simulink model "Step_12_TheEstimatedINVDynamicsMatricesCTC"  (R2020a)
settings: Solver=ode4  StartTime=0.0  StopTime=10  FixedStep=2e-3  RelTol=1e-3
model workspace (MATLAB code in the model file):
  | dhparams = [0   0   0.6   0;
  |             0   0   0     pi/2;
  |             0   0   0.5   0];
  | 
  | rrrRobot = rigidBodyTree('DataFormat', 'column', 'MaxNumBodies', 4);
  | 
  | bodyNames = {'link1', 'link2', 'link3'};
  | jointNames = {'joint1', 'joint2', 'joint3'};
  | parentNames = {'base', 'link1', 'link2'};
  | 
  | for i = 1:3
  |     body = rigidBody(bodyNames{i});
  |     joint = rigidBodyJoint(jointNames{i}, 'revolute');
  |     setFixedTransform(joint, dhparams(i,:), 'dh');
  |     body.Joint = joint;
  |     addBody(rrrRobot, body, parentNames{i});
  | end
  | 
  | tool = rigidBody('tool');
  | jointTool = rigidBodyJoint('fix_tip', 'fixed');
  | setFixedTransform(jointTool, eye(4));
  | tool.Joint = jointTool;
  | addBody(rrrRobot, tool, 'link3');
undefined symbols (not defined in the file or in its folder): X, Y, Z
libraries: sm_lib x34, nesl_utility x10
(part 2 of 2)

== matlab function Step_12_TheEstimatedINVDynamicsMatricesCTC/CTC/Estimated_C ==
  data: Q input; EstTau_C output; Qp input
function EstTau_C = Estimated_C(Q,Qp)
%#codegen

%    This function was generated by the Symbolic Math Toolbox version 8.5.
%    10-Jul-2026 17:57:50

q1 = Q(1,:);
q2 = Q(2,:);
q3 = Q(3,:);
qp1 = Qp(1,:);
qp2 = Qp(2,:);
qp3 = Qp(3,:);
EstTau_C = [qp1.*8.650376988596507e-4+tanh(qp1.*1.0e+2).*2.609157356257976e-3+cos(q2+q3).*(sin(q1).*(qp1.*qp2.*cos(q1)+qp1.*qp3.*cos(q1))-cos(q1).*(qp1.*qp2.*sin(q1)+qp1.*qp3.*sin(q1))).*2.289775576171808e-3-(qp2.*cos(q1).^2.*sin(q2)+qp2.*sin(q1).^2.*sin(q2)).*(qp2.*cos(q1).^2+qp2.*sin(q1).^2).*1.139509685512077e-2+(cos(q2+q3).*cos(q1).*(qp2.*cos(q1)+qp3.*cos(q1))+cos(q2+q3).*sin(q1).*(qp2.*sin(q1)+qp3.*sin(q1))).*(qp1.*cos(q2+q3)+sin(q2+q3).*sin(q1).*(qp2.*cos(q1)+qp3.*cos(q1))-sin(q2+q3).*cos(q1).*(qp2.*sin(q1)+qp3.*sin(q1))).*7.317250181898908e-3-sin(q2+q3).*(sin(q1).*(qp1.*qp2.*cos(q1)+qp1.*qp3.*cos(q1))-cos(q1).*(qp1.*qp2.*sin(q1)+qp1.*qp3.*sin(q1))).*5.967026219736011e-3-(sin(q2+q3).*cos(q1).*(qp2.*cos(q1)+qp3.*cos(q1))+sin(q2+q3).*sin(q1).*(qp2.*sin(q1)+qp3.*sin(q1))).*(qp1.*sin(q2+q3)-cos(q2+q3).*sin(q1).*(qp2.*cos(q1)+qp3.*cos(q1))+cos(q2+q3).*cos(q1).*(qp2.*sin(q1)+qp3.*sin(q1))).*7.317250181898908e-3+cos(q2+q3).*((cos(q1).*cos(q2).*(qp1.*qp2.*cos(q1)+qp1.*qp3.*cos(q1)))./2.0+(cos(q2).*sin(q1).*(qp1.*qp2.*sin(q1)+qp1.*qp3.*sin(q1)))./2.0+(qp1.*cos(q1).*cos(q2).*(qp2.*cos(q1)+qp3.*cos(q1)))./2.0+(qp1.*cos(q2).*sin(q1).*(qp2.*sin(q1)+qp3.*sin(q1)))./2.0).*3.199478300720183e-7+cos(q2).*(qp1.*qp2.*cos(q1).^2.*cos(q2)+qp1.*qp2.*cos(q2).*sin(q1).^2).*3.327734875462438e-3-(sin(q2+q3).*cos(q1).*(qp2.*cos(q1)+qp3.*cos(q1))+sin(q2+q3).*sin(q1).*(qp2.*sin(q1)+qp3.*sin(q1))).*(qp1.*cos(q2+q3)+sin(q2+q3).*sin(q1).*(qp2.*cos(q1)+qp3.*cos(q1))-sin(q2+q3).*cos(q1).*(qp2.*sin(q1)+qp3.*sin(q1))).*6.62632259505323e-2-(sin(q1).*(qp2.*sin(q1)+qp3.*sin(q1))+cos(q1).*(qp2.*cos(q1)+qp3.*cos(q1))).*(cos(q2+q3).*cos(q1).*(qp2.*cos(q1)+qp3.*cos(q1))+cos(q2+q3).*sin(q1).*(qp2.*sin(q1)+qp3.*sin(q1))).*5.967026219736011e-3-sin(q2+q3).*((cos(q1).*cos(q2).*(qp1.*qp2.*cos(q1)+qp1.*qp3.*cos(q1)))./2.0+(cos(q2).*sin(q1).*(qp1.*qp2.*sin(q1)+qp1.*qp3.*sin(q1)))./2.0+(qp1.*cos(q1).*cos(q2).*(qp2.*cos(q1)+qp3.*cos(q1)))./2.0+(qp1.*cos(q2).*sin(q1).*(qp2.*sin(q1)+qp3.*sin(q1)))./2.0).*3.000177417317213e-1+sin(q2).*(qp1.*qp2.*cos(q1).^2.*cos(q2)+qp1.*qp2.*cos(q2).*sin(q1).^2).*1.801758335412092e-2-cos(q2).*(qp1.*qp2.*cos(q1).^2.*sin(q2)+qp1.*qp2.*sin(q1).^2.*sin(q2)).*5.794502385359621e-1+cos(q2+q3).*(cos(q2+q3).*cos(q1).*(qp1.*qp2.*cos(q1)+qp1.*qp3.*cos(q1))+cos(q2+q3).*sin(q1).*(qp1.*qp2.*sin(q1)+qp1.*qp3.*sin(q1))).*7.317250181898908e-3-(sin(q1).*(qp2.*sin(q1)+qp3.*sin(q1))+cos(q1).*(qp2.*cos(q1)+qp3.*cos(q1))).*(sin(q2+q3).*cos(q1).*(qp2.*cos(q1)+qp3.*cos(q1))+sin(q2+q3).*sin(q1).*(qp2.*sin(q1)+qp3.*sin(q1))).*2.289775576171808e-3-sin(q2).*(qp1.*qp2.*cos(q1).^2.*sin(q2)+qp1.*qp2.*sin(q1).^2.*sin(q2)).*3.327734875462438e-3-cos(q2+q3).*(sin(q2+q3).*cos(q1).*(qp1.*qp2.*cos(q1)+qp1.*qp3.*cos(q1))+sin(q2+q3).*sin(q1).*(qp1.*qp2.*sin(q1)+qp1.*qp3.*sin(q1))).*6.62632259505323e-2-sin(q2+q3).*(sin(q2+q3).*cos(q1).*(qp1.*qp2.*cos(q1)+qp1.*qp3.*cos(q1))+sin(q2+q3).*sin(q1).*(qp1.*qp2.*sin(q1)+qp1.*qp3.*sin(q1))).*7.317250181898908e-3-(sin(q1).*(qp2.*cos(q1)+qp3.*cos(q1))-cos(q1).*(qp2.*sin(q1)+qp3.*sin(q1))).*(qp1.*sin(q2+q3)-cos(q2+q3).*sin(q1).*(qp2.*cos(q1)+qp3.*cos(q1))+cos(q2+q3).*cos(q1).*(qp2.*sin(q1)+qp3.*sin(q1))).*5.967026219736011e-3+(sin(q1).*(qp2.*cos(q1)+qp3.*cos(q1))-cos(q1).*(qp2.*sin(q1)+qp3.*sin(q1))).*(qp1.*cos(q2+q3)+sin(q2+q3).*sin(q1).*(qp2.*cos(q1)+qp3.*cos(q1))-sin(q2+q3).*cos(q1).*(qp2.*sin(q1)+qp3.*sin(q1))).*2.289775576171808e-3+(sin(q1).*(qp2.*sin(q1)+qp3.*sin(q1))+cos(q1).*(qp2.*cos(q1)+qp3.*cos(q1))).*(sin(q1).*(qp2.*cos(q1)+qp3.*cos(q1))-cos(q1).*(qp2.*sin(q1)+qp3.*sin(q1))).*8.244272995860623e-2+(qp2.*cos(q1).^2.*cos(q2)+qp2.*cos(q2).*sin(q1).^2).*(qp2.*cos(q1).^2+qp2.*sin(q1).^2).*7.881605381698013e-5-cos(q2+q3).*cos(q1).*(qp1.*((qp1.*cos(q2).*sin(q1))./2.0+(qp2.*cos(q1).*sin(q2))./2.0)+qp2.*((qp1.*cos(q1).*sin(q2))./2.0+(qp2.*cos(q2).*sin(q1))./2.0)-(qp2.*cos(q1)+qp3.*cos(q1)).*((cos(q2).*sin(q1).*(qp2.*cos(q1)+qp3.*cos(q1)))./2.0-(cos(q1).*cos(q2).*(qp2.*sin(q1)+qp3.*sin(q1)))./2.0)-(qp1.^2.*cos(q2).*sin(q1))./2.0).*3.000177417317213e-1-sin(q2+q3).*cos(q1).*(qp1.*((qp1.*cos(q2).*sin(q1))./2.0+(qp2.*cos(q1).*sin(q2))./2.0)+qp2.*((qp1.*cos(q1).*sin(q2))./2.0+(qp2.*cos(q2).*sin(q1))./2.0)-(qp2.*cos(q1)+qp3.*cos(q1)).*((cos(q2).*sin(q1).*(qp2.*cos(q1)+qp3.*cos(q1)))./2.0-(cos(q1).*cos(q2).*(qp2.*sin(q1)+qp3.*sin(q1)))./2.0)-(qp1.^2.*cos(q2).*sin(q1))./2.0).*3.199478300720183e-7+cos(q2+q3).*sin(q1).*((qp2.*sin(q1)+qp3.*sin(q1)).*((cos(q2).*sin(q1).*(qp2.*cos(q1)+qp3.*cos(q1)))./2.0-(cos(q1).*cos(q2).*(qp2.*sin(q1)+qp3.*sin(q1)))./2.0)+qp1.*((qp1.*cos(q1).*cos(q2))./2.0-(qp2.*sin(q1).*sin(q2))./2.0)+qp2.*((qp2.*cos(q1).*cos(q2))./2.0-(qp1.*sin(q1).*sin(q2))./2.0)-(qp1.^2.*cos(q1).*cos(q2))./2.0).*3.000177417317213e-1+qp1.*cos(q2).*(qp2.*cos(q1).^2.*cos(q2)+qp2.*cos(q2).*sin(q1).^2).*3.327734875462438e-3+sin(q2+q3).*sin(q1).*((qp2.*sin(q1)+qp3.*sin(q1)).*((cos(q2).*sin(q1).*(qp2.*cos(q1)+qp3.*cos(q1)))./2.0-(cos(q1).*cos(q2).*(qp2.*sin(q1)+qp3.*sin(q1)))./2.0)+qp1.*((qp1.*cos(q1).*cos(q2))./2.0-(qp2.*sin(q1).*sin(q2))./2.0)+qp2.*((qp2.*cos(q1).*cos(q2))./2.0-(qp1.*sin(q1).*sin(q2))./2.0)-(qp1.^2.*cos(q1).*cos(q2))./2.0).*3.199478300720183e-7+qp1.*sin(q2).*(qp2.*cos(q1).^2.*cos(q2)+qp2.*cos(q2).*sin(q1).^2).*1.801758335412092e-2-qp1.*cos(q2).*(qp2.*cos(q1).^2.*sin(q2)+qp2.*sin(q1).^2.*sin(q2)).*5.794502385359621e-1-qp1.*sin(q2).*(qp2.*cos(q1).^2.*sin(q2)+qp2.*sin(q1).^2.*sin(q2)).*3.327734875462438e-3;qp2.*(-1.309534126070689e-2)+tanh(qp2.*1.0e+2).*5.718358826714878e-3-sin(q1).*((cos(q2+q3).*(qp2.*cos(q1)+qp3.*cos(q1))-qp1.*sin(q2+q3).*sin(q1)).*(qp1.*cos(q2+q3)+sin(q2+q3).*sin(q1).*(qp2.*cos(q1)+qp3.*cos(q1))-sin(q2+q3).*cos(q1).*(qp2.*sin(q1)+qp3.*sin(q1)))-sin(q2+q3).*cos(q1).*(sin(q2+q3).*cos(q1).*(qp1.*qp2.*cos(q1)+qp1.*qp3.*cos(q1))+sin(q2+q3).*sin(q1).*(qp1.*qp2.*sin(q1)+qp1.*qp3.*sin(q1)))).*6.62632259505323e-2-sin(q1).*(-(sin(q1).*(qp2.*sin(q1)+qp3.*sin(q1))+cos(q1).*(qp2.*cos(q1)+qp3.*cos(q1))).*(sin(q2+q3).*(qp2.*cos(q1)+qp3.*cos(q1))+qp1.*cos(q2+q3).*sin(q1))+sin(q1).*(cos(q2+q3).*cos(q1).*(qp1.*qp2.*cos(q1)+qp1.*qp3.*cos(q1))+cos(q2+q3).*sin(q1).*(qp1.*qp2.*sin(q1)+qp1.*qp3.*sin(q1)))+qp1.*cos(q1).*(qp1.*sin(q2+q3)-cos(q2+q3).*sin(q1).*(qp2.*cos(q1)+qp3.*cos(q1))+cos(q2+q3).*cos(q1).*(qp2.*sin(q1)+qp3.*sin(q1)))+cos(q2+q3).*cos(q1).*(sin(q1).*(qp1.*qp2.*cos(q1)+qp1.*qp3.*cos(q1))-cos(q1).*(qp1.*qp2.*sin(q1)+qp1.*qp3.*sin(q1)))).*5.967026219736011e-3-cos(q1).*(-cos(q1).*(qp1.*qp2.*cos(q1).^2.*cos(q2)+qp1.*qp2.*cos(q2).*sin(q1).^2)+(qp1.*cos(q1).*cos(q2)-qp2.*sin(q1).*sin(q2)).*(qp2.*cos(q1).^2+qp2.*sin(q1).^2)+qp1.^2.*sin(q1).*sin(q2)).*7.881605381698013e-5+cos(q2+q3).*((qp2.*sin(q1)+qp3.*sin(q1)).*((cos(q2).*(qp2.*sin(q1)+qp3.*sin(q1)))./2.0+(qp1.*cos(q1).*sin(q2))./2.0)-cos(q1).*(qp1.*((qp1.*cos(q1).*cos(q2))./2.0-(qp2.*sin(q1).*sin(q2))./2.0)+qp2.*((qp2.*cos(q1).*cos(q2))./2.0-(qp1.*sin(q1).*sin(q2))./2.0))-sin(q1).*(qp1.*((qp1.*cos(q2).*sin(q1))./2.0+(qp2.*cos(q1).*sin(q2))./2.0)+qp2.*((qp1.*cos(q1).*sin(q2))./2.0+(qp2.*cos(q2).*sin(q1))./2.0))+(qp2.*cos(q1)+qp3.*cos(q1)).*((cos(q2).*(qp2.*cos(q1)+qp3.*cos(q1)))./2.0-(qp1.*sin(q1).*sin(q2))./2.0)-(sin(q1).*sin(q2).*(qp1.*qp2.*cos(q1)+qp1.*qp3.*cos(q1)))./2.0+(cos(q1).*sin(q2).*(qp1.*qp2.*sin(q1)+qp1.*qp3.*sin(q1)))./2.0).*3.199478300720183e-7+cos(q1).*((cos(q2+q3).*(qp2.*sin(q1)+qp3.*sin(q1))+qp1.*sin(q2+q3).*cos(q1)).*(qp1.*cos(q2+q3)+sin(q2+q3).*sin(q1).*(qp2.*cos(q1)+qp3.*cos(q1))-sin(q2+q3).*cos(q1).*(qp2.*sin(q1)+qp3.*sin(q1)))-sin(q2+q3).*sin(q1).*(sin(q2+q3).*cos(q1).*(qp1.*qp2.*cos(q1)+qp1.*qp3.*cos(q1))+sin(q2+q3).*sin(q1).*(qp1.*qp2.*sin(q1)+qp1.*qp3.*sin(q1)))).*6.62632259505323e-2-cos(q1).*((sin(q1).*(qp2.*sin(q1)+qp3.*sin(q1))+cos(q1).*(qp2.*cos(q1)+qp3.*cos(q1))).*(sin(q2+q3).*(qp2.*sin(q1)+qp3.*sin(q1))-qp1.*cos(q2+q3).*cos(q1))+cos(q1).*(cos(q2+q3).*cos(q1).*(qp1.*qp2.*cos(q1)+qp1.*qp3.*cos(q1))+cos(q2+q3).*sin(q1).*(qp1.*qp2.*sin(q1)+qp1.*qp3.*sin(q1)))-qp1.*sin(q1).*(qp1.*sin(q2+q3)-cos(q2+q3).*sin(q1).*(qp2.*cos(q1)+qp3.*cos(q1))+cos(q2+q3).*cos(q1).*(qp2.*sin(q1)+qp3.*sin(q1)))-cos(q2+q3).*sin(q1).*(sin(q1).*(qp1.*qp2.*cos(q1)+qp1.*qp3.*cos(q1))-cos(q1).*(qp1.*qp2.*sin(q1)+qp1.*qp3.*sin(q1)))).*5.967026219736011e-3-cos(q1).*(-(qp1.*cos(q1).*sin(q2)+qp2.*cos(q2).*sin(q1)).*(qp2.*cos(q1).^2+qp2.*sin(q1).^2)+cos(q1).*(qp1.*qp2.*cos(q1).^2.*sin(q2)+qp1.*qp2.*sin(q1).^2.*sin(q2))+qp1.^2.*cos(q2).*sin(q1)).*1.139509685512077e-2+sin(q1).*(sin(q1).*(qp1.*qp2.*cos(q1).^2.*cos(q2)+qp1.*qp2.*cos(q2).*sin(q1).^2)-(qp1.*cos(q2).*sin(q1)+qp2.*cos(q1).*sin(q2)).*(qp2.*cos(q1).^2+qp2.*sin(q1).^2)+qp1.^2.*cos(q1).*sin(q2)).*7.881605381698013e-5-sin(q2+q3).*((qp2.*sin(q1)+qp3.*sin(q1)).*((cos(q2).*(qp2.*sin(q1)+qp3.*sin(q1)))./2.0+(qp1.*cos(q1).*sin(q2))./2.0)-cos(q1).*(qp1.*((qp1.*cos(q1).*cos(q2))./2.0-(qp2.*sin(q1).*sin(q2))./2.0)+qp2.*((qp2.*cos(q1).*cos(q2))./2.0-(qp1.*sin(q1).*sin(q2))./2.0))-sin(q1).*(qp1.*((qp1.*cos(q2).*sin(q1))./2.0+(qp2.*cos(q1).*sin(q2))./2.0)+qp2.*((qp1.*cos(q1).*sin(q2))./2.0+(qp2.*cos(q2).*sin(q1))./2.0))+(qp2.*cos(q1)+qp3.*cos(q1)).*((cos(q2).*(qp2.*cos(q1)+qp3.*cos(q1)))./2.0-(qp1.*sin(q1).*sin(q2))./2.0)-(sin(q1).*sin(q2).*(qp1.*qp2.*cos(q1)+qp1.*qp3.*cos(q1)))./2.0+(cos(q1).*sin(q2).*(qp1.*qp2.*sin(q1)+qp1.*qp3.*sin(q1)))./2.0).*3.000177417317213e-1-sin(q1).*(qp1.*cos(q2).*(qp1.*cos(q2).*sin(q1)+qp2.*cos(q1).*sin(q2))+cos(q1).*sin(q2).*(qp1.*qp2.*cos(q1).^2.*cos(q2)+qp1.*qp2.*cos(q2).*sin(q1).^2)+qp1.*sin(q2).*(qp2.*cos(q1).*cos(q2)-qp1.*sin(q1).*sin(q2))+cos(q1).*cos(q2).*(qp1.*qp2.*cos(q1).^2.*sin(q2)+qp1.*qp2.*sin(q1).^2.*sin(q2))).*3.327734875462438e-3-sin(q1).*((sin(q2+q3).*(qp2.*cos(q1)+qp3.*cos(q1))+qp1.*cos(q2+q3).*sin(q1)).*(qp1.*cos(q2+q3)+sin(q2+q3).*sin(q1).*(qp2.*cos(q1)+qp3.*cos(q1))-sin(q2+q3).*cos(q1).*(qp2.*sin(q1)+qp3.*sin(q1)))+(cos(q2+q3).*(qp2.*cos(q1)+qp3.*cos(q1))-qp1.*sin(q2+q3).*sin(q1)).*(qp1.*sin(q2+q3)-cos(q2+q3).*sin(q1).*(qp2.*cos(q1)+qp3.*cos(q1))+cos(q2+q3).*cos(q1).*(qp2.*sin(q1)+qp3.*sin(q1)))+sin(q2+q3).*cos(q1).*(cos(q2+q3).*cos(q1).*(qp1.*qp2.*cos(q1)+qp1.*qp3.*cos(q1))+cos(q2+q3).*sin(q1).*(qp1.*qp2.*sin(q1)+qp1.*qp3.*sin(q1)))+cos(q2+q3).*cos(q1).*(sin(q2+q3).*cos(q1).*(qp1.*qp2.*cos(q1)+qp1.*qp3.*cos(q1))+sin(q2+q3).*sin(q1).*(qp1.*qp2.*sin(q1)+qp1.*qp3.*sin(q1)))).*7.317250181898908e-3-sin(q1).*((qp2.*cos(q1).*cos(q2)-qp1.*sin(q1).*sin(q2)).*(qp2.*cos(q1).^2+qp2.*sin(q1).^2)+sin(q1).*(qp1.*qp2.*cos(q1).^2.*sin(q2)+qp1.*qp2.*sin(q1).^2.*sin(q2))-qp1.^2.*cos(q1).*cos(q2)).*1.139509685512077e-2+cos(q2+q3).*cos(q1).^2.*2.940173868970869+cos(q1).*(-qp1.*cos(q2).*(qp1.*cos(q1).*cos(q2)-qp2.*sin(q1).*sin(q2))+qp1.*sin(q2).*(qp1.*cos(q1).*sin(q2)+qp2.*cos(q2).*sin(q1))+sin(q1).*sin(q2).*(qp1.*qp2.*cos(q1).^2.*cos(q2)+qp1.*qp2.*cos(q2).*sin(q1).^2)+cos(q2).*sin(q1).*(qp1.*qp2.*cos(q1).^2.*sin(q2)+qp1.*qp2.*sin(q1).^2.*sin(q2))).*3.327734875462438e-3+cos(q2+q3).*sin(q1).^2.*2.940173868970869+sin(q2+q3).*cos(q1).^2.*3.135488734705779e-6-sin(q1).*((sin(q1).*(qp2.*sin(q1)+qp3.*sin(q1))+cos(q1).*(qp2.*cos(q1)+qp3.*cos(q1))).*(cos(q2+q3).*(qp2.*cos(q1)+qp3.*cos(q1))-qp1.*sin(q2+q3).*sin(q1))+sin(q1).*(sin(q2+q3).*cos(q1).*(qp1.*qp2.*cos(q1)+qp1.*qp3.*cos(q1))+sin(q2+q3).*sin(q1).*(qp1.*qp2.*sin(q1)+qp1.*qp3.*sin(q1)))-qp1.*cos(q1).*(qp1.*cos(q2+q3)+sin(q2+q3).*sin(q1).*(qp2.*cos(q1)+qp3.*cos(q1))-sin(q2+q3).*cos(q1).*(qp2.*sin(q1)+qp3.*sin(q1)))+sin(q2+q3).*cos(q1).*(sin(q1).*(qp1.*qp2.*cos(q1)+qp1.*qp3.*cos(q1))-cos(q1).*(qp1.*qp2.*sin(q1)+qp1.*qp3.*sin(q1)))).*2.289775576171808e-3+sin(q2+q3).*sin(q1).^2.*3.135488734705779e-6+cos(q1).*((sin(q1).*(qp2.*sin(q1)+qp3.*sin(q1))+cos(q1).*(qp2.*cos(q1)+qp3.*cos(q1))).*(cos(q2+q3).*(qp2.*sin(q1)+qp3.*sin(q1))+qp1.*sin(q2+q3).*cos(q1))-cos(q1).*(sin(q2+q3).*cos(q1).*(qp1.*qp2.*cos(q1)+qp1.*qp3.*cos(q1))+sin(q2+q3).*sin(q1).*(qp1.*qp2.*sin(q1)+qp1.*qp3.*sin(q1)))+sin(q2+q3).*sin(q1).*(sin(q1).*(qp1.*qp2.*cos(q1)+qp1.*qp3.*cos(q1))-cos(q1).*(qp1.*qp2.*sin(q1)+qp1.*qp3.*sin(q1)))-qp1.*sin(q1).*(qp1.*cos(q2+q3)+sin(q2+q3).*sin(q1).*(qp2.*cos(q1)+qp3.*cos(q1))-sin(q2+q3).*cos(q1).*(qp2.*sin(q1)+qp3.*sin(q1)))).*2.289775576171808e-3+cos(q1).*((cos(q2+q3).*(qp2.*sin(q1)+qp3.*sin(q1))+qp1.*sin(q2+q3).*cos(q1)).*(qp1.*sin(q2+q3)-cos(q2+q3).*sin(q1).*(qp2.*cos(q1)+qp3.*cos(q1))+cos(q2+q3).*cos(q1).*(qp2.*sin(q1)+qp3.*sin(q1)))+(sin(q2+q3).*(qp2.*sin(q1)+qp3.*sin(q1))-qp1.*cos(q2+q3).*cos(q1)).*(qp1.*cos(q2+q3)+sin(q2+q3).*sin(q1).*(qp2.*cos(q1)+qp3.*cos(q1))-sin(q2+q3).*cos(q1).*(qp2.*sin(q1)+qp3.*sin(q1)))+sin(q2+q3).*sin(q1).*(cos(q2+q3).*cos(q1).*(qp1.*qp2.*cos(q1)+qp1.*qp3.*cos(q1))+cos(q2+q3).*sin(q1).*(qp1.*qp2.*sin(q1)+qp1.*qp3.*sin(q1)))+cos(q2+q3).*sin(q1).*(sin(q2+q3).*cos(q1).*(qp1.*qp2.*cos(q1)+qp1.*qp3.*cos(q1))+sin(q2+q3).*sin(q1).*(qp1.*qp2.*sin(q1)+qp1.*qp3.*sin(q1)))).*7.317250181898908e-3-cos(q1).*(cos(q2).*sin(q1).*(qp1.*qp2.*cos(q1).^2.*cos(q2)+qp1.*qp2.*cos(q2).*sin(q1).^2)+qp1.*sin(q2).*(qp1.*cos(q1).*cos(q2)-qp2.*sin(q1).*sin(q2))).*1.801758335412092e-2+sin(q1).*(cos(q1).*cos(q2).*(qp1.*qp2.*cos(q1).^2.*cos(q2)+qp1.*qp2.*cos(q2).*sin(q1).^2)-qp1.*sin(q2).*(qp1.*cos(q2).*sin(q1)+qp2.*cos(q1).*sin(q2))).*1.801758335412092e-2+cos(q1).*(cos(q1).*(sin(q1).*(qp1.*qp2.*cos(q1)+qp1.*qp3.*cos(q1))-cos(q1).*(qp1.*qp2.*sin(q1)+qp1.*qp3.*sin(q1)))-qp1.*sin(q1).*(sin(q1).*(qp2.*sin(q1)+qp3.*sin(q1))+cos(q1).*(qp2.*cos(q1)+qp3.*cos(q1)))).*8.244272995860623e-2+sin(q1).*(sin(q1).*(sin(q1).*(qp1.*qp2.*cos(q1)+qp1.*qp3.*cos(q1))-cos(q1).*(qp1.*qp2.*sin(q1)+qp1.*qp3.*sin(q1)))+qp1.*cos(q1).*(sin(q1).*(qp2.*sin(q1)+qp3.*sin(q1))+cos(q1).*(qp2.*cos(q1)+qp3.*cos(q1)))).*8.244272995860623e-2+cos(q1).*(qp1.*cos(q2).*(qp1.*cos(q1).*sin(q2)+qp2.*cos(q2).*sin(q1))-sin(q1).*sin(q2).*(qp1.*qp2.*cos(q1).^2.*sin(q2)+qp1.*qp2.*sin(q1).^2.*sin(q2))).*5.794502385359621e-1-sin(q1).*(qp1.*cos(q2).*(qp2.*cos(q1).*cos(q2)-qp1.*sin(q1).*sin(q2))-cos(q1).*sin(q2).*(qp1.*qp2.*cos(q1).^2.*sin(q2)+qp1.*qp2.*sin(q1).^2.*sin(q2))).*5.794502385359621e-1+cos(q2+q3).*cos(q1).*(((cos(q1).*sin(q2).*(qp2.*cos(q1)+qp3.*cos(q1)))./2.0+(sin(q1).*sin(q2).*(qp2.*sin(q1)+qp3.*sin(q1)))./2.0).*(qp2.*cos(q1)+qp3.*cos(q1))-cos(q1).*((qp2.^2.*sin(q2))./2.0+4.9e+1./5.0)+qp1.*((cos(q2).*(qp2.*sin(q1)+qp3.*sin(q1)))./2.0+(qp1.*cos(q1).*sin(q2))./2.0)-(cos(q2).*(qp1.*qp2.*sin(q1)+qp1.*qp3.*sin(q1)))./2.0).*3.000177417317213e-1+sin(q2+q3).*cos(q1).*(((cos(q1).*sin(q2).*(qp2.*cos(q1)+qp3.*cos(q1)))./2.0+(sin(q1).*sin(q2).*(qp2.*sin(q1)+qp3.*sin(q1)))./2.0).*(qp2.*cos(q1)+qp3.*cos(q1))-cos(q1).*((qp2.^2.*sin(q2))./2.0+4.9e+1./5.0)+qp1.*((cos(q2).*(qp2.*sin(q1)+qp3.*sin(q1)))./2.0+(qp1.*cos(q1).*sin(q2))./2.0)-(cos(q2).*(qp1.*qp2.*sin(q1)+qp1.*qp3.*sin(q1)))./2.0).*3.199478300720183e-7+cos(q2+q3).*sin(q1).*(((cos(q1).*sin(q2).*(qp2.*cos(q1)+qp3.*cos(q1)))./2.0+(sin(q1).*sin(q2).*(qp2.*sin(q1)+qp3.*sin(q1)))./2.0).*(qp2.*sin(q1)+qp3.*sin(q1))-qp1.*((cos(q2).*(qp2.*cos(q1)+qp3.*cos(q1)))./2.0-(qp1.*sin(q1).*sin(q2))./2.0)-sin(q1).*((qp2.^2.*sin(q2))./2.0+4.9e+1./5.0)+(cos(q2).*(qp1.*qp2.*cos(q1)+qp1.*qp3.*cos(q1)))./2.0).*3.000177417317213e-1+sin(q2+q3).*sin(q1).*(((cos(q1).*sin(q2).*(qp2.*cos(q1)+qp3.*cos(q1)))./2.0+(sin(q1).*sin(q2).*(qp2.*sin(q1)+qp3.*sin(q1)))./2.0).*(qp2.*sin(q1)+qp3.*sin(q1))-qp1.*((cos(q2).*(qp2.*cos(q1)+qp3.*cos(q1)))./2.0-(qp1.*sin(q1).*sin(q2))./2.0)-sin(q1).*((qp2.^2.*sin(q2))./2.0+4.9e+1./5.0)+(cos(q2).*(qp1.*qp2.*cos(q1)+qp1.*qp3.*cos(q1)))./2.0).*3.199478300720183e-7;qp3.*1.645741718765586e-4+tanh(qp3.*1.0e+2).*1.118634117620773e-3-sin(q1).*((cos(q2+q3).*(qp2.*cos(q1)+qp3.*cos(q1))-qp1.*sin(q2+q3).*sin(q1)).*(qp1.*cos(q2+q3)+sin(q2+q3).*sin(q1).*(qp2.*cos(q1)+qp3.*cos(q1))-sin(q2+q3).*cos(q1).*(qp2.*sin(q1)+qp3.*sin(q1)))-sin(q2+q3).*cos(q1).*(sin(q2+q3).*cos(q1).*(qp1.*qp2.*cos(q1)+qp1.*qp3.*cos(q1))+sin(q2+q3).*sin(q1).*(qp1.*qp2.*sin(q1)+qp1.*qp3.*sin(q1)))).*6.62632259505323e-2-sin(q1).*(-(sin(q1).*(qp2.*sin(q1)+qp3.*sin(q1))+cos(q1).*(qp2.*cos(q1)+qp3.*cos(q1))).*(sin(q2+q3).*(qp2.*cos(q1)+qp3.*cos(q1))+qp1.*cos(q2+q3).*sin(q1))+sin(q1).*(cos(q2+q3).*cos(q1).*(qp1.*qp2.*cos(q1)+qp1.*qp3.*cos(q1))+cos(q2+q3).*sin(q1).*(qp1.*qp2.*sin(q1)+qp1.*qp3.*sin(q1)))+qp1.*cos(q1).*(qp1.*sin(q2+q3)-cos(q2+q3).*sin(q1).*(qp2.*cos(q1)+qp3.*cos(q1))+cos(q2+q3).*cos(q1).*(qp2.*sin(q1)+qp3.*sin(q1)))+cos(q2+q3).*cos(q1).*(sin(q1).*(qp1.*qp2.*cos(q1)+qp1.*qp3.*cos(q1))-cos(q1).*(qp1.*qp2.*sin(q1)+qp1.*qp3.*sin(q1)))).*5.967026219736011e-3+cos(q1).*((cos(q2+q3).*(qp2.*sin(q1)+qp3.*sin(q1))+qp1.*sin(q2+q3).*cos(q1)).*(qp1.*cos(q2+q3)+sin(q2+q3).*sin(q1).*(qp2.*cos(q1)+qp3.*cos(q1))-sin(q2+q3).*cos(q1).*(qp2.*sin(q1)+qp3.*sin(q1)))-sin(q2+q3).*sin(q1).*(sin(q2+q3).*cos(q1).*(qp1.*qp2.*cos(q1)+qp1.*qp3.*cos(q1))+sin(q2+q3).*sin(q1).*(qp1.*qp2.*sin(q1)+qp1.*qp3.*sin(q1)))).*6.62632259505323e-2-cos(q1).*((sin(q1).*(qp2.*sin(q1)+qp3.*sin(q1))+cos(q1).*(qp2.*cos(q1)+qp3.*cos(q1))).*(sin(q2+q3).*(qp2.*sin(q1)+qp3.*sin(q1))-qp1.*cos(q2+q3).*cos(q1))+cos(q1).*(cos(q2+q3).*cos(q1).*(qp1.*qp2.*cos(q1)+qp1.*qp3.*cos(q1))+cos(q2+q3).*sin(q1).*(qp1.*qp2.*sin(q1)+qp1.*qp3.*sin(q1)))-qp1.*sin(q1).*(qp1.*sin(q2+q3)-cos(q2+q3).*sin(q1).*(qp2.*cos(q1)+qp3.*cos(q1))+cos(q2+q3).*cos(q1).*(qp2.*sin(q1)+qp3.*sin(q1)))-cos(q2+q3).*sin(q1).*(sin(q1).*(qp1.*qp2.*cos(q1)+qp1.*qp3.*cos(q1))-cos(q1).*(qp1.*qp2.*sin(q1)+qp1.*qp3.*sin(q1)))).*5.967026219736011e-3-sin(q1).*((sin(q2+q3).*(qp2.*cos(q1)+qp3.*cos(q1))+qp1.*cos(q2+q3).*sin(q1)).*(qp1.*cos(q2+q3)+sin(q2+q3).*sin(q1).*(qp2.*cos(q1)+qp3.*cos(q1))-sin(q2+q3).*cos(q1).*(qp2.*sin(q1)+qp3.*sin(q1)))+(cos(q2+q3).*(qp2.*cos(q1)+qp3.*cos(q1))-qp1.*sin(q2+q3).*sin(q1)).*(qp1.*sin(q2+q3)-cos(q2+q3).*sin(q1).*(qp2.*cos(q1)+qp3.*cos(q1))+cos(q2+q3).*cos(q1).*(qp2.*sin(q1)+qp3.*sin(q1)))+sin(q2+q3).*cos(q1).*(cos(q2+q3).*cos(q1).*(qp1.*qp2.*cos(q1)+qp1.*qp3.*cos(q1))+cos(q2+q3).*sin(q1).*(qp1.*qp2.*sin(q1)+qp1.*qp3.*sin(q1)))+cos(q2+q3).*cos(q1).*(sin(q2+q3).*cos(q1).*(qp1.*qp2.*cos(q1)+qp1.*qp3.*cos(q1))+sin(q2+q3).*sin(q1).*(qp1.*qp2.*sin(q1)+qp1.*qp3.*sin(q1)))).*7.317250181898908e-3+cos(q2+q3).*cos(q1).^2.*2.940173868970869+cos(q2+q3).*sin(q1).^2.*2.940173868970869+sin(q2+q3).*cos(q1).^2.*3.135488734705779e-6-sin(q1).*((sin(q1).*(qp2.*sin(q1)+qp3.*sin(q1))+cos(q1).*(qp2.*cos(q1)+qp3.*cos(q1))).*(cos(q2+q3).*(qp2.*cos(q1)+qp3.*cos(q1))-qp1.*sin(q2+q3).*sin(q1))+sin(q1).*(sin(q2+q3).*cos(q1).*(qp1.*qp2.*cos(q1)+qp1.*qp3.*cos(q1))+sin(q2+q3).*sin(q1).*(qp1.*qp2.*sin(q1)+qp1.*qp3.*sin(q1)))-qp1.*cos(q1).*(qp1.*cos(q2+q3)+sin(q2+q3).*sin(q1).*(qp2.*cos(q1)+qp3.*cos(q1))-sin(q2+q3).*cos(q1).*(qp2.*sin(q1)+qp3.*sin(q1)))+sin(q2+q3).*cos(q1).*(sin(q1).*(qp1.*qp2.*cos(q1)+qp1.*qp3.*cos(q1))-cos(q1).*(qp1.*qp2.*sin(q1)+qp1.*qp3.*sin(q1)))).*2.289775576171808e-3+sin(q2+q3).*sin(q1).^2.*3.135488734705779e-6+cos(q1).*((sin(q1).*(qp2.*sin(q1)+qp3.*sin(q1))+cos(q1).*(qp2.*cos(q1)+qp3.*cos(q1))).*(cos(q2+q3).*(qp2.*sin(q1)+qp3.*sin(q1))+qp1.*sin(q2+q3).*cos(q1))-cos(q1).*(sin(q2+q3).*cos(q1).*(qp1.*qp2.*cos(q1)+qp1.*qp3.*cos(q1))+sin(q2+q3).*sin(q1).*(qp1.*qp2.*sin(q1)+qp1.*qp3.*sin(q1)))+sin(q2+q3).*sin(q1).*(sin(q1).*(qp1.*qp2.*cos(q1)+qp1.*qp3.*cos(q1))-cos(q1).*(qp1.*qp2.*sin(q1)+qp1.*qp3.*sin(q1)))-qp1.*sin(q1).*(qp1.*cos(q2+q3)+sin(q2+q3).*sin(q1).*(qp2.*cos(q1)+qp3.*cos(q1))-sin(q2+q3).*cos(q1).*(qp2.*sin(q1)+qp3.*sin(q1)))).*2.289775576171808e-3+cos(q1).*((cos(q2+q3).*(qp2.*sin(q1)+qp3.*sin(q1))+qp1.*sin(q2+q3).*cos(q1)).*(qp1.*sin(q2+q3)-cos(q2+q3).*sin(q1).*(qp2.*cos(q1)+qp3.*cos(q1))+cos(q2+q3).*cos(q1).*(qp2.*sin(q1)+qp3.*sin(q1)))+(sin(q2+q3).*(qp2.*sin(q1)+qp3.*sin(q1))-qp1.*cos(q2+q3).*cos(q1)).*(qp1.*cos(q2+q3)+sin(q2+q3).*sin(q1).*(qp2.*cos(q1)+qp3.*cos(q1))-sin(q2+q3).*cos(q1).*(qp2.*sin(q1)+qp3.*sin(q1)))+sin(q2+q3).*sin(q1).*(cos(q2+q3).*cos(q1).*(qp1.*qp2.*cos(q1)+qp1.*qp3.*cos(q1))+cos(q2+q3).*sin(q1).*(qp1.*qp2.*sin(q1)+qp1.*qp3.*sin(q1)))+cos(q2+q3).*sin(q1).*(sin(q2+q3).*cos(q1).*(qp1.*qp2.*cos(q1)+qp1.*qp3.*cos(q1))+sin(q2+q3).*sin(q1).*(qp1.*qp2.*sin(q1)+qp1.*qp3.*sin(q1)))).*7.317250181898908e-3-cos(q2+q3).*(cos(q1).*(qp1.*((qp1.*cos(q1).*cos(q2))./2.0-(qp2.*sin(q1).*sin(q2))./2.0)+qp2.*((qp2.*cos(q1).*cos(q2))./2.0-(qp1.*sin(q1).*sin(q2))./2.0))+sin(q1).*(qp1.*((qp1.*cos(q2).*sin(q1))./2.0+(qp2.*cos(q1).*sin(q2))./2.0)+qp2.*((qp1.*cos(q1).*sin(q2))./2.0+(qp2.*cos(q2).*sin(q1))./2.0))).*3.199478300720183e-7+sin(q2+q3).*(cos(q1).*(qp1.*((qp1.*cos(q1).*cos(q2))./2.0-(qp2.*sin(q1).*sin(q2))./2.0)+qp2.*((qp2.*cos(q1).*cos(q2))./2.0-(qp1.*sin(q1).*sin(q2))./2.0))+sin(q1).*(qp1.*((qp1.*cos(q2).*sin(q1))./2.0+(qp2.*cos(q1).*sin(q2))./2.0)+qp2.*((qp1.*cos(q1).*sin(q2))./2.0+(qp2.*cos(q2).*sin(q1))./2.0))).*3.000177417317213e-1+cos(q1).*(cos(q1).*(sin(q1).*(qp1.*qp2.*cos(q1)+qp1.*qp3.*cos(q1))-cos(q1).*(qp1.*qp2.*sin(q1)+qp1.*qp3.*sin(q1)))-qp1.*sin(q1).*(sin(q1).*(qp2.*sin(q1)+qp3.*sin(q1))+cos(q1).*(qp2.*cos(q1)+qp3.*cos(q1)))).*8.244272995860623e-2+sin(q1).*(sin(q1).*(sin(q1).*(qp1.*qp2.*cos(q1)+qp1.*qp3.*cos(q1))-cos(q1).*(qp1.*qp2.*sin(q1)+qp1.*qp3.*sin(q1)))+qp1.*cos(q1).*(sin(q1).*(qp2.*sin(q1)+qp3.*sin(q1))+cos(q1).*(qp2.*cos(q1)+qp3.*cos(q1)))).*8.244272995860623e-2-cos(q2+q3).*cos(q1).^2.*((qp2.^2.*sin(q2))./2.0+4.9e+1./5.0).*3.000177417317213e-1-cos(q2+q3).*sin(q1).^2.*((qp2.^2.*sin(q2))./2.0+4.9e+1./5.0).*3.000177417317213e-1-sin(q2+q3).*cos(q1).^2.*((qp2.^2.*sin(q2))./2.0+4.9e+1./5.0).*3.199478300720183e-7-sin(q2+q3).*sin(q1).^2.*((qp2.^2.*sin(q2))./2.0+4.9e+1./5.0).*3.199478300720183e-7];

== matlab function Step_12_TheEstimatedINVDynamicsMatricesCTC/CTC/Estimated_G ==
  data: Q input; EstTau_G output
function EstTau_G = Estimated_G(Q)
%#codegen

%    This function was generated by the Symbolic Math Toolbox version 8.5.
%    10-Jul-2026 17:57:50

q1 = Q(1,:);
q2 = Q(2,:);
q3 = Q(3,:);
EstTau_G = [0.0;cos(q2+q3).*cos(q1).^2.*(-2.940173868970869)-cos(q2+q3).*sin(q1).^2.*2.940173868970869-sin(q2+q3).*cos(q1).^2.*3.135488734705779e-6-sin(q2+q3).*sin(q1).^2.*3.135488734705779e-6-cos(q1).^2.*cos(q2).*1.348632571564392e+1-cos(q2).*sin(q1).^2.*1.348632571564392e+1+cos(q1).^2.*sin(q2).*1.037455707524711e-2+sin(q1).^2.*sin(q2).*1.037455707524711e-2;cos(q2+q3).*cos(q1).^2.*(-2.940173868970869)-cos(q2+q3).*sin(q1).^2.*2.940173868970869-sin(q2+q3).*cos(q1).^2.*3.135488734705779e-6-sin(q2+q3).*sin(q1).^2.*3.135488734705779e-6];

== matlab function Step_12_TheEstimatedINVDynamicsMatricesCTC/CTC/Estimated_M ==
  data: Q input; EstTau_M output
function EstTau_M = Estimated_M(Q)
%#codegen

%    This function was generated by the Symbolic Math Toolbox version 8.5.
%    10-Jul-2026 17:57:49

q1 = Q(1,:);
q2 = Q(2,:);
q3 = Q(3,:);
EstTau_M = reshape([cos(q2+q3).^2.*6.62632259505323e-2+cos(q2).*sin(q2).*6.655469750924875e-3+cos(q2).^2.*5.794502385359621e-1+sin(q2).^2.*1.801758335412092e-2+cos(q2+q3).*sin(q2+q3).*1.463450036379782e-2+cos(q2+q3).*cos(q1).^2.*cos(q2).*3.000177417317213e-1+cos(q2+q3).*cos(q2).*sin(q1).^2.*3.000177417317213e-1+sin(q2+q3).*cos(q1).^2.*cos(q2).*3.199478300720183e-7+sin(q2+q3).*cos(q2).*sin(q1).^2.*3.199478300720183e-7,sin(q1).*(cos(q2+q3).^2.*cos(q1)-sin(q2+q3).^2.*cos(q1)).*7.317250181898908e-3-cos(q1).*(cos(q2+q3).^2.*sin(q1)-sin(q2+q3).^2.*sin(q1)).*7.317250181898908e-3+cos(q2+q3).*cos(q1).^2.*2.289775576171808e-3+cos(q2+q3).*sin(q1).^2.*2.289775576171808e-3-sin(q2+q3).*cos(q1).^2.*5.967026219736011e-3-sin(q2+q3).*sin(q1).^2.*5.967026219736011e-3+cos(q1).^2.*cos(q2).*1.139509685512077e-2+cos(q2).*sin(q1).^2.*1.139509685512077e-2+cos(q1).^2.*sin(q2).*7.881605381698013e-5+sin(q1).*(cos(q1).*cos(q2).^2-cos(q1).*sin(q2).^2).*3.327734875462438e-3+sin(q1).^2.*sin(q2).*7.881605381698013e-5-cos(q1).*(cos(q2).^2.*sin(q1)-sin(q1).*sin(q2).^2).*3.327734875462438e-3,sin(q1).*(cos(q2+q3).^2.*cos(q1)-sin(q2+q3).^2.*cos(q1)).*7.317250181898908e-3-cos(q1).*(cos(q2+q3).^2.*sin(q1)-sin(q2+q3).^2.*sin(q1)).*7.317250181898908e-3+cos(q2+q3).*cos(q1).^2.*2.289775576171808e-3+cos(q2+q3).*sin(q1).^2.*2.289775576171808e-3-sin(q2+q3).*cos(q1).^2.*5.967026219736011e-3-sin(q2+q3).*sin(q1).^2.*5.967026219736011e-3,cos(q2).*(cos(q1).^2+sin(q1).^2).*1.139509685512077e-2+sin(q2).*(cos(q1).^2+sin(q1).^2).*7.881605381698013e-5+cos(q2+q3).*(cos(q1).^2+sin(q1).^2).*2.289775576171808e-3-sin(q2+q3).*(cos(q1).^2+sin(q1).^2).*5.967026219736011e-3,cos(q2+q3).*(cos(q1).^2.*sin(q2)+sin(q1).^2.*sin(q2)).*(-3.199478300720183e-7)+cos(q1).^2.*(cos(q1).^2+sin(q1).^2).*6.704456229949877e-1+sin(q2+q3).*(cos(q1).^2.*sin(q2)+sin(q1).^2.*sin(q2)).*3.000177417317213e-1+sin(q1).^2.*(cos(q1).^2+sin(q1).^2).*6.704456229949877e-1+cos(q2+q3).*cos(q1).^2.*cos(q2).*3.000177417317213e-1+cos(q2+q3).*cos(q2).*sin(q1).^2.*3.000177417317213e-1+sin(q2+q3).*cos(q1).^2.*cos(q2).*3.199478300720183e-7+sin(q2+q3).*cos(q2).*sin(q1).^2.*3.199478300720183e-7,cos(q2+q3).*((cos(q1).^2.*sin(q2))./2.0+(sin(q1).^2.*sin(q2))./2.0).*(-3.199478300720183e-7)+cos(q1).^2.*(cos(q1).^2+sin(q1).^2).*8.244272995860623e-2+sin(q2+q3).*((cos(q1).^2.*sin(q2))./2.0+(sin(q1).^2.*sin(q2))./2.0).*3.000177417317213e-1+sin(q1).^2.*(cos(q1).^2+sin(q1).^2).*8.244272995860623e-2+cos(q2+q3).*cos(q1).^2.*cos(q2).*1.500088708658606e-1+cos(q2+q3).*cos(q2).*sin(q1).^2.*1.500088708658606e-1+sin(q2+q3).*cos(q1).^2.*cos(q2).*1.599739150360091e-7+sin(q2+q3).*cos(q2).*sin(q1).^2.*1.599739150360091e-7,cos(q2+q3).*(cos(q1).^2+sin(q1).^2).*2.289775576171808e-3-sin(q2+q3).*(cos(q1).^2+sin(q1).^2).*5.967026219736011e-3,cos(q2+q3).*((cos(q1).^2.*sin(q2))./2.0+(sin(q1).^2.*sin(q2))./2.0).*(-3.199478300720183e-7)+cos(q1).^2.*(cos(q1).^2+sin(q1).^2).*8.244272995860623e-2+sin(q2+q3).*((cos(q1).^2.*sin(q2))./2.0+(sin(q1).^2.*sin(q2))./2.0).*3.000177417317213e-1+sin(q1).^2.*(cos(q1).^2+sin(q1).^2).*8.244272995860623e-2+cos(q2+q3).*cos(q1).^2.*cos(q2).*1.500088708658606e-1+cos(q2+q3).*cos(q2).*sin(q1).^2.*1.500088708658606e-1+sin(q2+q3).*cos(q1).^2.*cos(q2).*1.599739150360091e-7+sin(q2+q3).*cos(q2).*sin(q1).^2.*1.599739150360091e-7,cos(q1).^2.*(cos(q1).^2+sin(q1).^2).*8.244272995860623e-2+sin(q1).^2.*(cos(q1).^2+sin(q1).^2).*8.244272995860623e-2],[3,3]);
